simulink model "HW2a"  (Simulink 8.5)
settings: Solver=ode45  StartTime=0.0  StopTime=25  MaxStep=0.1  MinStep=0.0001  RelTol=1e-3  AbsTol=1e-3
settings Model: Creator=Hybrid Pederson  LastModifiedBy=ccpc50
settings DataIOCC: SaveOutput=off  SaveTime=off
settings OptimizationCC: InitFltsAndDblsToZero=on
settings DebuggingCC: SaveWithParameterizedLinksMsg=none  SolverPrmCheckMsg=warning  FcnCallInpInsideContextMsg=UseLocalSettings
settings GRTTargetCC: TargetFcnLib=ansi_tfl_tmw.mat

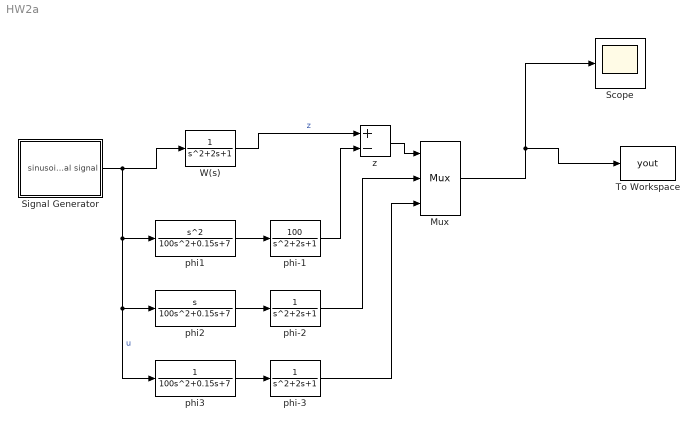
== system HW2a ==
  Mux : Mux  Inputs=3
  Scope : Scope
      settings: TickLabels=on  ShowLegends=on  TimeRange=50  YMin=-20.000000  YMax=20.000000
  Signal Generator : Subsystem
      mask Display: plot(sin([0.0:0.1:6.3])
  To Workspace : ToWorkspace  VariableName=yout
      settings: MaxDataPoints=5000
  W(s) : TransferFcn
  phi-1 : TransferFcn  Numerator=[100]
  phi-2 : TransferFcn
  phi-3 : TransferFcn
  phi1 : TransferFcn  Numerator=[1 0 0]  Denominator=[100 0.15 7]
  phi2 : TransferFcn  Numerator=[1 0]  Denominator=[100 0.15 7]
  phi3 : TransferFcn  Denominator=[100 0.15 7]
  z : Sum  Inputs=+-
  wires:
  Mux/1 -> To Workspace/1, Scope/1
  Signal Generator/1(sinusoidal signal) -> phi3/1, phi2/1, phi1/1, W(s)/1  "u"
  phi2/1 -> phi-2/1
  phi1/1 -> phi-1/1
  phi3/1 -> phi-3/1
  phi-1/1 -> z/2
  phi-2/1 -> Mux/2
  W(s)/1 -> z/1  "z"
  z/1 -> Mux/1
  phi-3/1 -> Mux/3

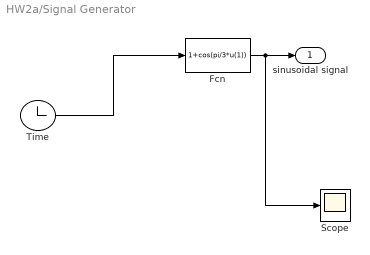
== system HW2a/Signal Generator ==
  Fcn : Fcn  Expr=1+cos(pi/3*u(1))
      mask Display: disp('A sin(wt+p)')
  Scope : Scope
  Time : Clock
  sinusoidal signal : Outport
  wires:
  Time/1 -> Fcn/1
  Fcn/1 -> Scope/1, sinusoidal signal/1
